simulink model "servo_PID_n_sim"  (R2020a)
settings: Solver=ode5  StartTime=0.0  StopTime=30  FixedStep=0.02  RelTol=1e-3  EnableMultiTasking=on
PreLoadFcn:
  | load servo_chstat
values from neighbouring files (symbols this model uses):
  K = [0.06  0.0 0.0125]    [servo_start.m]
undefined symbols (not defined in the file or in its folder): pwm, vpwm
settings Model: Creator=Administrator  LastModifiedBy=inteco
settings DataIOCC: LimitDataPoints=on  SaveFormat=Array  SignalLoggingSaveFormat=ModelDataLogs  ReturnWorkspaceOutputs=off  SignalLoggingName=sigsOut
settings OptimizationCC: ExpressionDepthLimit=2147483647  InitFltsAndDblsToZero=on  LifeSpan=inf
settings DebuggingCC: SaveWithParameterizedLinksMsg=none  UnderspecifiedInitializationDetection=Classic  MergeDetectMultiDrivingBlocksExec=none  SignalResolutionControl=TryResolveAllWithWarning  MultiTaskDSMMsg=warning  MultiTaskCondExecSysMsg=none  FcnCallInpInsideContextMsg=warning  StateNameClashWarn=warning  PregeneratedLibrarySubsystemCodeDiagnostic=none  SFUnexpectedBacktrackingDiag=warning  SFNoUnconditionalDefaultTransitionDiag=warning  SFExecutionAtInitializationDiag=none  ArithmeticOperatorsInVariantConditions=warning
settings HardwareCC: ProdBitPerPointer=32  ProdBitPerSizeT=32  ProdBitPerPtrDiffT=32  ProdLargestAtomicFloat=None  ProdIntDivRoundTo=Undefined  ProdEndianess=Unspecified  ProdWordSize=32  ProdHWDeviceType=32-bit Generic  TargetBitPerPointer=64  TargetBitPerSizeT=64  TargetBitPerPtrDiffT=64  TargetLongLongMode=on  TargetIntDivRoundTo=Zero  TargetEndianess=LittleEndian  TargetWordSize=64  TargetHWDeviceType=MATLAB Host  ProdEqTarget=off
settings ModelReferenceCC: PropagateSignalLabelsOutOfModel=off
settings SFSimCC: SimUseLocalCustomCode=off  CustomCodeUndefinedFunction=UseInterfaceOnly
settings RTWCC: RTWUseLocalCustomCode=off
settings CodeAppCC: StateflowObjectComments=on
settings GRTTargetCC: TargetFcnLib=ansi_tfl_tmw.mat  TargetLangStandard=C89/C90 (ANSI)  CombineOutputUpdateFcns=off  GRTInterface=on
settings ConfigComp: CovMetricSettings=dw  CovHtmlReporting=on  CovSaveCumulativeToWorkspaceVar=on  CovSaveSingleToWorkspaceVar=on  CovExternalEMLEnable=off  CovSFcnEnable=off

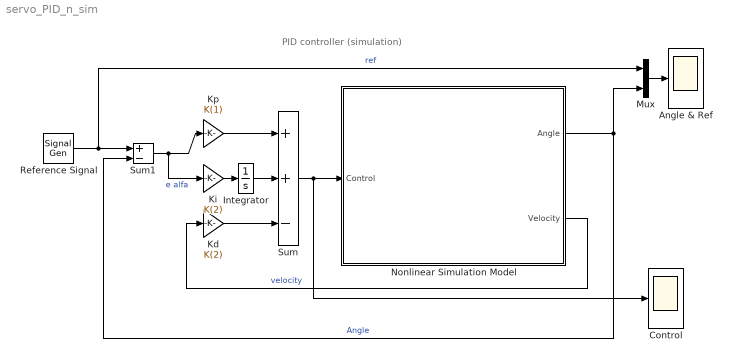
== system servo_PID_n_sim ==
  note: PID controller (simulation)
  Angle & Ref : Scope
  Control : Scope
  Integrator : Integrator
  Kd : Gain  Gain=K(2)  SaturateOnIntegerOverflow=on  OutDataTypeStr=Inherit: Same as input  ParamDataTypeStr=Inherit: Same as input
  Ki : Gain  Gain=K(2)  SaturateOnIntegerOverflow=on  OutDataTypeStr=Inherit: Same as input  ParamDataTypeStr=Inherit: Same as input
  Kp : Gain  Gain=K(1)  SaturateOnIntegerOverflow=on  OutDataTypeStr=Inherit: Same as input  ParamDataTypeStr=Inherit: Same as input
  Mux : Mux  Inputs=2
  Nonlinear Simulation Model : Subsystem  mask{x0=[0 0], c_n=206, Parameter3=[vpwm pwm]}
      mask prompts: x0 "Initial conditions [angle velocity]"; c_n "Gain c"; Parameter3 "Static characteristic [velocity control]"
      mask Help:
      | The parameters necessary for this block are:
      | 1. Static characteristic implemented as Look-up table block (vectors vpwm and pwm),
      | 2. gain  - c ,
      | 3. Initial conditions - x0,
      | Refer to 3.2 section in User's Manual.
      | 
      | 
      | The model preloads the default static characteristic from servo_chstat.mat file.
      | To change default characteristic a user should load a new vpwm and pwm vectors or
      | replace servo_chstat.mat file.
      mask Display: image(imread('Servo_m.JPG'))
  "Reference Signal " : SignalGenerator  WaveForm=square  Amplitude=pi*25/2  Frequency=0.05
  Sum : Sum  Inputs=++-  InputSameDT=on  SaturateOnIntegerOverflow=on  OutDataTypeStr=Inherit: Same as first input
  Sum1 : Sum  Inputs=+-  InputSameDT=on  SaturateOnIntegerOverflow=on  OutDataTypeStr=Inherit: Same as first input
  wires:
  Kp/1 -> Sum/1
  Sum1/1 -> Kp/1, Ki/1  "e alfa"
  "Reference Signal "/1 -> Sum1/1, Mux/1  "ref"
  Mux/1 -> Angle & Ref/1
  Sum/1 -> Nonlinear Simulation Model/1(Control), Control/1
  Nonlinear Simulation Model/1(Angle) -> Mux/2, Sum1/2  "Angle"
  Nonlinear Simulation Model/2(Velocity) -> Kd/1  "velocity"
  Ki/1 -> Integrator/1
  Kd/1 -> Sum/3
  Integrator/1 -> Sum/2

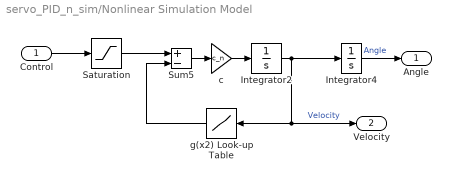
== system servo_PID_n_sim/Nonlinear Simulation Model ==
  Control : Inport
  Integrator2 : Integrator  InitialCondition=x0(2)
  Integrator4 : Integrator  InitialCondition=x0(1)
  Saturation : Saturate  UpperLimit=1  LowerLimit=-1
  Sum5 : Sum  Inputs=+-  InputSameDT=on  SaturateOnIntegerOverflow=on  OutDataTypeStr=Inherit: Same as first input
  c : Gain  Gain=c_n  SaturateOnIntegerOverflow=on  OutDataTypeStr=Inherit: Same as input  ParamDataTypeStr=Inherit: Same as input
  g(x2) Look-up Table : Lookup  InputValues=vpwm  Table=pwm  SaturateOnIntegerOverflow=on
  Angle : Outport  InitialOutput=0  VectorParamsAs1DForOutWhenUnconnected=off
  Velocity : Outport  Port=2  InitialOutput=0  VectorParamsAs1DForOutWhenUnconnected=off
  wires:
  Saturation/1 -> Sum5/1
  Control/1 -> Saturation/1
  c/1 -> Integrator2/1
  Integrator4/1 -> Angle/1  "Angle"
  Integrator2/1 -> g(x2) Look-up Table/1, Velocity/1, Integrator4/1  "Velocity"
  g(x2) Look-up Table/1 -> Sum5/2
  Sum5/1 -> c/1
